simulink model "CSWI_test22"  (Simulink 7.8)
settings: Solver=FixedStepDiscrete  StartTime=0.0  StopTime=t_sim  FixedStep=1/6400  RelTol=1e-3
undefined symbols (not defined in the file or in its folder): sigbuilder_block
settings Model: Creator=schukin  LastModifiedBy=nikonenok

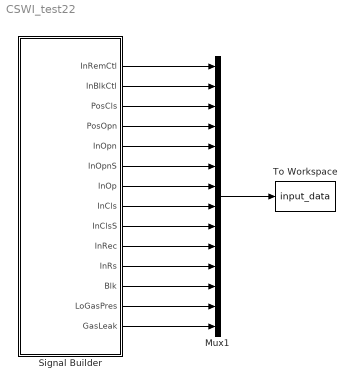
== system CSWI_test22 ==
  Mux1 : Mux  Inputs=14
  Signal Builder : Subsystem  Tag=STV Subsys  LoadFcn=sigbuilder_block('load',[539.25 81 547.5 585 ]);  StartFcn=sigbuilder_block('start');  StopFcn=sigbuilder_block('stop');  ClipboardFcn=sigbuilder_block('clipboard');  mask(Sigbuilder block){}
      mask help: Simulink:masks:SigbuilderBlock_MD
      mask init:
      | if ~strcmp(get_param(bdroot(gcbh),'SimulationStatus'),'stopped') tuvar = sigbuilder_block('maskInit'); end
      settings: CopyFcn=sigbuilder_block('copy');  DeleteFcn=sigbuilder_block('delete');  ModelCloseFcn=sigbuilder_block('modelClose');  PreSaveFcn=sigbuilder_block('preSave');  NameChangeFcn=sigbuilder_block('namechange');  OpenFcn=sigbuilder_block('open',[539.25 81 547.5 585 ]);  CloseFcn=sigbuilder_block('close');
      mask Display: plot(0, 0, 100, 100,[2, 2, 32, 32, 2], [68, 8, 8, 68, 68],[32, 2], [38, 38], [32, 19, 2],[53, 60, 44], [32, 17, 17, 2],[16, 16, 31, 31]);txt = getActiveGroup(gcbh);text(2, 100, txt,'verticalAlignment', 'top');
  To Workspace : ToWorkspace  VariableName=input_data  SampleTime=-1  SaveFormat=Structure With Time
  wires:
  Mux1/1 -> To Workspace/1
  Signal Builder/1(InRemCtl) -> Mux1/1
  Signal Builder/2(InBlkCtl) -> Mux1/2
  Signal Builder/3(PosCls) -> Mux1/3
  Signal Builder/4(PosOpn) -> Mux1/4
  Signal Builder/5(InOpn) -> Mux1/5
  Signal Builder/6(InOpnS) -> Mux1/6
  Signal Builder/7(InOp) -> Mux1/7
  Signal Builder/8(InCls) -> Mux1/8
  Signal Builder/9(InClsS) -> Mux1/9
  Signal Builder/10(InRec) -> Mux1/10
  Signal Builder/11(InRs) -> Mux1/11
  Signal Builder/12(Blk) -> Mux1/12
  Signal Builder/13(LoGasPres) -> Mux1/13
  Signal Builder/14(GasLeak) -> Mux1/14

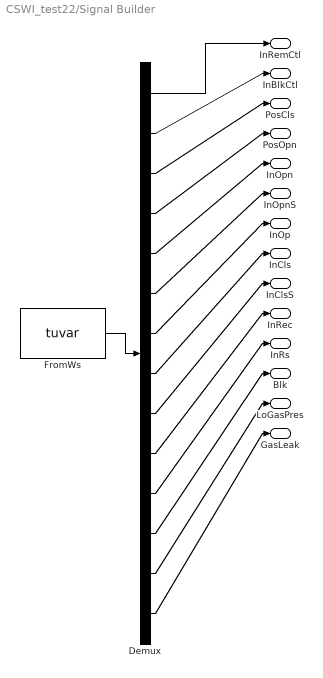
== system CSWI_test22/Signal Builder ==
  Demux : Demux  Tag=STV Demux  Outputs=14
  FromWs : FromWorkspace  Tag=STV FromWs  VariableName=tuvar  SampleTime=0  SigBuilderData=DataTag0  VnvData=DataTag1
      SigBuilderData=|
      | common.afterFinalStr = 'Extrapolate'
      | common.sampleTime = 0
      | dataSet.timeRange = [0 5]
      | dataSet.name = 'Group 1'
      | sbobj.Groups.Name = 'Group 1'
      | sbobj.Groups.Signals(1).Name = 'InRemCtl'
      | sbobj.Groups.Signals(1).XData = [0 1.2 1.2 2.5 2.5 5]
      | sbobj.Groups.Signals(1).YData = [0 0 1 1 0 0]
      | sbobj.Groups.Signals(2).Name = 'InBlkCtl'
      | sbobj.Groups.Signals(2).XData = [0 1 1.25 5]
      | sbobj.Groups.Signals(2).YData = [0 0 0 0]
      | sbobj.Groups.Signals(3).Name = 'PosCls'
      | sbobj.Groups.Signals(3).XData = [0 1.5 1.75 5]
      | sbobj.Groups.Signals(3).YData = [0 0 0 0]
      | sbobj.Groups.Signals(4).Name = 'PosOpn'
      | sbobj.Groups.Signals(4).XData = [0 0.51 1 5]
      | sbobj.Groups.Signals(4).YData = [0 0 0 0]
      | sbobj.Groups.Signals(5).Name = 'InOpn'
      | sbobj.Groups.Signals(5).XData = [0 0.51 1 5]
      | sbobj.Groups.Signals(5).YData = [0 0 0 0]
      | sbobj.Groups.Signals(6).Name = 'InOpnS'
      | sbobj.Groups.Signals(6).XData = [0 0.51 1 5]
      | sbobj.Groups.Signals(6).YData = [0 0 0 0]
      | sbobj.Groups.Signals(7).Name = 'InOp'
      | sbobj.Groups.Signals(7).XData = [0 0.51 1 5]
      | sbobj.Groups.Signals(7).YData = [0 0 0 0]
      | sbobj.Groups.Signals(8).Name = 'InCls'
      | sbobj.Groups.Signals(8).XData = [0 1.6 1.6 1.7 1.7 5]
      | sbobj.Groups.Signals(8).YData = [0 0 1 1 0 0]
      | sbobj.Groups.Signals(9).Name = 'InClsS'
      | sbobj.Groups.Signals(9).XData = [0 0.51 1 5]
      | sbobj.Groups.Signals(9).YData = [0 0 0 0]
      | sbobj.Groups.Signals(10).Name = 'InRec'
      | sbobj.Groups.Signals(10).XData = [0 0.51 1 5]
      | sbobj.Groups.Signals(10).YData = [0 0 0 0]
      | sbobj.Groups.Signals(11).Name = 'InRs'
      | sbobj.Groups.Signals(11).XData = [0 2.4 2.4 2.5 2.5 5]
      | sbobj.Groups.Signals(11).YData = [0 0 1 1 0 0]
      | sbobj.Groups.Signals(12).Name = 'Blk'
      | sbobj.Groups.Signals(12).XData = [0 1.55 1.55 1.72 1.72 5]
      | sbobj.Groups.Signals(12).YData = [0 0 1 1 0 0]
      | sbobj.Groups.Signals(13).Name = 'LoGasPres'
      | sbobj.Groups.Signals(13).XData = [0 0.51 1 5]
      | sbobj.Groups.Signals(13).YData = [0 0 0 0]
      | sbobj.Groups.Signals(14).Name = 'GasLeak'
      | sbobj.Groups.Signals(14).XData = [0 0.51 1 5]
      | sbobj.Groups.Signals(14).YData = [0 0 0 0]
      | sbobj.Groups.TimeRange = [0 5]
  InRemCtl : Outport  Tag=STV Outport
  InBlkCtl : Outport  Tag=STV Outport  Port=2
  PosCls : Outport  Tag=STV Outport  Port=3
  PosOpn : Outport  Tag=STV Outport  Port=4
  InOpn : Outport  Tag=STV Outport  Port=5
  InOpnS : Outport  Tag=STV Outport  Port=6
  InOp : Outport  Tag=STV Outport  Port=7
  InCls : Outport  Tag=STV Outport  Port=8
  InClsS : Outport  Tag=STV Outport  Port=9
  InRec : Outport  Tag=STV Outport  Port=10
  InRs : Outport  Tag=STV Outport  Port=11
  Blk : Outport  Tag=STV Outport  Port=12
  LoGasPres : Outport  Tag=STV Outport  Port=13
  GasLeak : Outport  Tag=STV Outport  Port=14
  wires:
  Demux/1 -> InRemCtl/1
  FromWs/1 -> Demux/1
  Demux/2 -> InBlkCtl/1
  Demux/3 -> PosCls/1
  Demux/4 -> PosOpn/1
  Demux/5 -> InOpn/1
  Demux/6 -> InOpnS/1
  Demux/7 -> InOp/1
  Demux/8 -> InCls/1
  Demux/9 -> InClsS/1
  Demux/10 -> InRec/1
  Demux/11 -> InRs/1
  Demux/12 -> Blk/1
  Demux/13 -> LoGasPres/1
  Demux/14 -> GasLeak/1
